simulink model "controllore_simulink"  (Simulink 8.3)
settings: Solver=ode45  StartTime=0.0  StopTime=30  RelTol=1e-3
values from neighbouring files (symbols this model uses):
  D1 = 1    [controllore.m]
  D2 = 1    [controllore.m]
libraries: cstblocks x2, simulink x1
settings Model: Creator=matdo  LastModifiedBy=matdo
settings DataIOCC: SignalLoggingSaveFormat=Dataset
settings DebuggingCC: UnderspecifiedInitializationDetection=Simplified  StateNameClashWarn=none
settings GRTTargetCC: CombineOutputUpdateFcns=on  GRTInterface=off

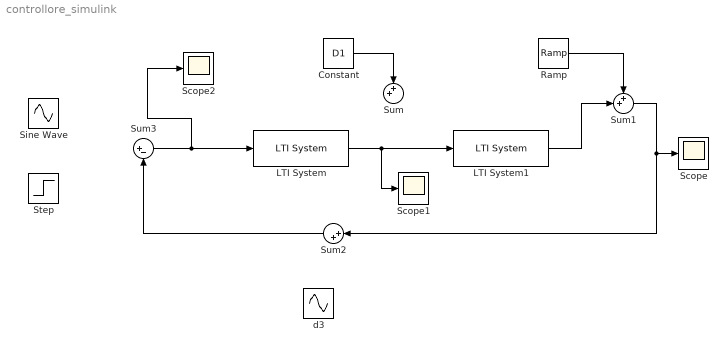
== system controllore_simulink ==
  Constant : Constant  Value=D1
  LTI System : cstblocks/LTI System  sys=Ci  IC=[]
  LTI System1 : cstblocks/LTI System  sys=F  IC=[]
  Ramp : simulink/Sources/Ramp  slope=D2  start=0  X0=0
  Scope : Scope
  Scope1 : Scope
  Scope2 : Scope
      settings: SaveName=ScopeData2
  Sine Wave : Sin  Frequency=0.5  SampleTime=0
  Step : Step  Time=0  SampleTime=0
  Sum : Sum  Inputs=++|
  Sum1 : Sum  Inputs=++|
  Sum2 : Sum  Inputs=|++
  Sum3 : Sum  Inputs=|+-
  d3 : Sin  Frequency=1000  SampleTime=0
  wires:
  Constant/1 -> Sum/1
  Ramp/1 -> Sum1/1
  Sum2/1 -> Sum3/2
  Sum3/1 -> Scope2/1, LTI System/1
  LTI System/1 -> Scope1/1, LTI System1/1
  LTI System1/1 -> Sum1/2
  Sum1/1 -> Sum2/1, Scope/1
